simulink model "Wnch"  (R2014b)
settings: Solver=ode45  StartTime=0.0  StopTime=10  MaxStep=0.001  MinStep=0.0001  RelTol=1e-3
values from neighbouring files (symbols this model uses):
  K = 195    [kurs.m]
  T1 = 0.018    [kurs.m]
  T2 = 0.18    [kurs.m]
libraries: simulink x1
settings Model: Creator=Игорь  LastModifiedBy=Игорь

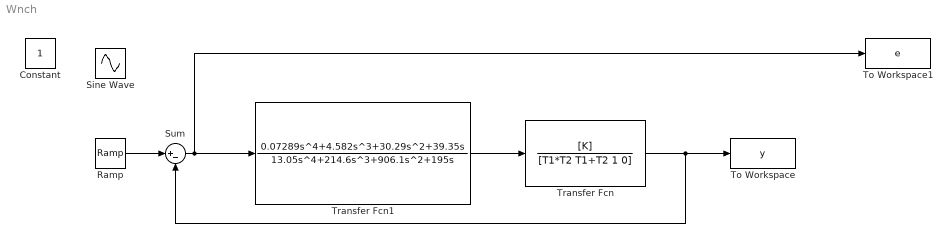
== system Wnch ==
  Constant : Constant
  Ramp : simulink/Sources/Ramp  slope=1.1  start=0  X0=0
  Sine Wave : Sin  Amplitude=4.8394  Frequency=0.2273  SampleTime=0
  Sum : Sum  Inputs=|+-
  To Workspace : ToWorkspace  VariableName=y  SaveFormat=Timeseries  SampleTime=-1
  To Workspace1 : ToWorkspace  VariableName=e  SaveFormat=Timeseries  SampleTime=-1
  Transfer Fcn : TransferFcn  Numerator=[K]  Denominator=[T1*T2 T1+T2 1 0]
  Transfer Fcn1 : TransferFcn  Numerator=[0.07289 4.582 30.29 39.35 0]  Denominator=[13.05 214.6 906.1 195 0]
  wires:
  Transfer Fcn/1 -> To Workspace/1, Sum/2
  Sum/1 -> To Workspace1/1, Transfer Fcn1/1
  Transfer Fcn1/1 -> Transfer Fcn/1
  Ramp/1 -> Sum/1
